simulink model "simulink_playground"  (R2019a)
settings: Solver=VariableStepAuto  StartTime=0.0  StopTime=0.1  MinStep=0.1  RelTol=1e-3
undefined symbols (not defined in the file or in its folder): MM
settings Model: Creator=carne  LastModifiedBy=carne
settings DataIOCC: ReturnWorkspaceOutputs=off
settings DebuggingCC: ArithmeticOperatorsInVariantConditions=warning

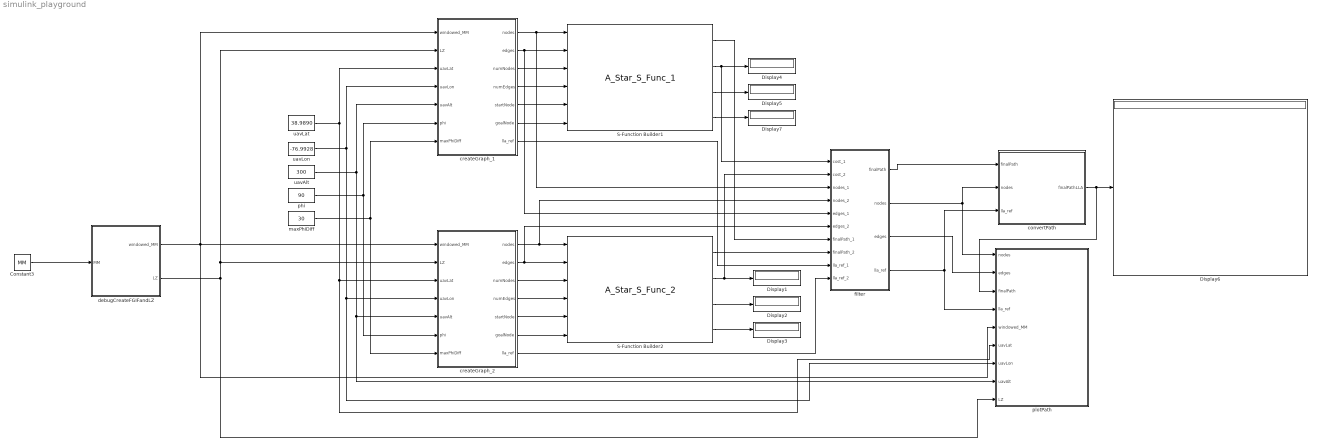
== system simulink_playground ==
  Constant3 : Constant  Value=MM
  Display{1..7} (7 alike) : Display
      Display1 settings: Format=decimal (Stored Integer)
      Display4 settings: Format=decimal (Stored Integer)
      Display6 settings: Format=decimal (Stored Integer)
  S-Function Builder1 : S-Function  InitFcn=try, set_param(gcb,'FunctionName','A_Star_S_Func_1'), end  FunctionName=A_Star_S_Func_1  SFunctionModules=A_Star_S_Func_1_wrapper  SFunctionDeploymentMode=off  EnableBusSupport=off  mask(S-Function Builder){}
      mask help: Simulink:masks:SFunctionBuilder_MD
      mask init:
      | val = [[.9  0.75 0.75 1 1 .9 .9 1]',[1 1 0.75 0.75 .9 .9 1 .9]'];try , sys = get_param(gcb,'SfunBuilderFcnName');if isempty(sys), sys = get_param(gcb,'FunctionName'); end,catch, sys = get_param(gcb,'FunctionName'); end
      settings: CopyFcn=set_param(gcbh,'LinkStatus','none')  PreSaveFcn=try, set_param(gcb,'FunctionName','A_Star_S_Func_1'), end  OpenFcn=sfunctionwizard(gcbh)
      mask Display: plot(val(:,1),val(:,2)),disp(sys), port_label('input',1,'nodeArray'), port_label('input',2,'edgeArray'), port_label('input',3,'numNodesPtr'), port_label('input',4,'numEdgesPtr'), port_label('input',5,'startNodePtr'), port_label('input',6,'goalNodePtr'), port_label('output',1,'finalPath'), port_label('output',2,'finalPathCost'), port_label('output',3,'numNodesCheck'), port_label('output',4,'numEdgesCheck')
  S-Function Builder2 : S-Function  InitFcn=try, set_param(gcb,'FunctionName','A_Star_S_Func_2'), end  FunctionName=A_Star_S_Func_2  SFunctionModules=A_Star_S_Func_2_wrapper  SFunctionDeploymentMode=off  EnableBusSupport=off  mask(S-Function Builder){}
      mask help: Simulink:masks:SFunctionBuilder_MD
      mask init: same as simulink_playground/S-Function Builder1
      settings: CopyFcn=set_param(gcbh,'LinkStatus','none')  PreSaveFcn=try, set_param(gcb,'FunctionName','A_Star_S_Func_2'), end  OpenFcn=sfunctionwizard(gcbh)
      mask Display: plot(val(:,1),val(:,2)),disp(sys), port_label('input',1,'nodeArray'), port_label('input',2,'edgeArray'), port_label('input',3,'numNodesPtr'), port_label('input',4,'numEdgesPtr'), port_label('input',5,'startNodePtr'), port_label('input',6,'goalNodePtr'), port_label('output',1,'finalPath'), port_label('output',2,'finalPathCost'), port_label('output',3,'numNodesCheck'), port_label('output',4,'numEdgesCheck')
  convertPath : MATLAB Function  TreatAsAtomicUnit=on
  createGraph_1 : MATLAB Function  TreatAsAtomicUnit=on
  createGraph_2 : MATLAB Function  TreatAsAtomicUnit=on
  debugCreateFGIFandLZ : MATLAB Function  TreatAsAtomicUnit=on
  filter : MATLAB Function  TreatAsAtomicUnit=on
  maxPhiDiff : Constant  Value=30
  phi : Constant  Value=90
  plotPath : MATLAB Function  TreatAsAtomicUnit=on
  uavAlt : Constant  Value=300
  uavLat : Constant  Value=38.9890
  uavLon : Constant  Value=-76.9928
  wires:
  createGraph_1/4(numEdges) -> S-Function Builder1/4
  createGraph_1/3(numNodes) -> S-Function Builder1/3
  createGraph_1/1(nodes) -> filter/3(nodes_1), S-Function Builder1/1
  createGraph_1/2(edges) -> filter/5(edges_1), S-Function Builder1/2
  S-Function Builder1/3 -> Display5/1
  S-Function Builder1/2 -> filter/1(cost_1), Display4/1
  uavAlt/1 -> plotPath/8(uavAlt), createGraph_2/5(uavAlt), createGraph_1/5(uavAlt)
  Constant3/1 -> debugCreateFGIFandLZ/1(MM)
  debugCreateFGIFandLZ/2(LZ) -> createGraph_1/2(LZ), createGraph_2/2(LZ), plotPath/9(LZ)
  S-Function Builder1/4 -> Display7/1
  uavLon/1 -> plotPath/7(uavLon), createGraph_2/4(uavLon), createGraph_1/4(uavLon)
  uavLat/1 -> plotPath/6(uavLat), createGraph_2/3(uavLat), createGraph_1/3(uavLat)
  phi/1 -> createGraph_2/6(phi), createGraph_1/6(phi)
  maxPhiDiff/1 -> createGraph_2/7(maxPhiDiff), createGraph_1/7(maxPhiDiff)
  convertPath/1(finalPathLLA) -> plotPath/3(finalPath), Display6/1
  debugCreateFGIFandLZ/1(windowed_MM) -> plotPath/5(windowed_MM), createGraph_1/1(windowed_MM), createGraph_2/1(windowed_MM)
  createGraph_1/5(startNode) -> S-Function Builder1/5
  createGraph_1/6(goalNode) -> S-Function Builder1/6
  createGraph_2/4(numEdges) -> S-Function Builder2/4
  createGraph_2/3(numNodes) -> S-Function Builder2/3
  createGraph_2/2(edges) -> filter/6(edges_2), S-Function Builder2/2
  createGraph_2/1(nodes) -> filter/4(nodes_2), S-Function Builder2/1
  createGraph_2/5(startNode) -> S-Function Builder2/5
  createGraph_2/6(goalNode) -> S-Function Builder2/6
  S-Function Builder2/3 -> Display2/1
  S-Function Builder2/2 -> filter/2(cost_2), Display1/1
  S-Function Builder2/4 -> Display3/1
  filter/1(finalPath) -> convertPath/1(finalPath)
  filter/2(nodes) -> convertPath/2(nodes), plotPath/1(nodes)
  filter/4(lla_ref) -> convertPath/3(lla_ref), plotPath/4(lla_ref)
  filter/3(edges) -> plotPath/2(edges)
  S-Function Builder2/1 -> filter/8(finalPath_2)
  S-Function Builder1/1 -> filter/7(finalPath_1)
  createGraph_2/7(lla_ref) -> filter/10(lla_ref_2)
  createGraph_1/7(lla_ref) -> filter/9(lla_ref_1)

== matlab function simulink_playground/plotPath ==
  data: nodes input; edges input; finalPath input; lla_ref input; windowed_MM input; uavLat input; uavLon input; uavAlt input; LZ input
function plotPath(nodes, edges, finalPath, lla_ref, windowed_MM, uavLat, uavLon, uavAlt, LZ)

    % setup altitude array for 3D matrix
    altDelta = 20.0;
    
    % convert altitude to meters
    uavAlt = uavAlt * 0.3048; % convert alt to meters
    altDelta = altDelta * 0.3048; % convert to meters
    
    % instantiate goal node variables
    goalNode = 0;
    goalNodeRow = 0;
    goalNodeCol = 0;
    
    numLzRows = max(LZ(:,1)) - min(LZ(:,1)) + 1;
    numLzCols = max(LZ(:,2)) - min(LZ(:,2)) + 1;
    
    % set the goal node row and column based on the orientation of the LZ
    if numLzRows > numLzCols
        goalNodeRow = min(LZ(:,1)); % right now pick one end of the LZ
        goalNodeCol = min(LZ(:,2)) + floor(numLzCols / 2); % pick the center column
    elseif numLzRows < numLzCols
        goalNodeCol = min(LZ(:,2)); % right now pick one end of the LZ
        goalNodeRow = min(LZ(:,1)) + floor(numLzRows / 2); % pick the center column
    end
    
    %% Create Altitude Array
    
    % setup altitude array for 3D matrix
    % currently this goes from UAV alt to zero, need to update this to
    % limit the lower altitude to the elevation of the landing strip
%     lzAlt = windowed_MM(goalNodeRow, goalNodeCol, 2);
%     altArray = [uavAlt:-altDelta:lzAlt];
%     if altArray(end) > lzAlt
%         altArray = [altArray, lzAlt];
%     end
%     [~, heightNum] = size(altArray);

    % WGS84 ellipsoid constants:
    a = 6378137;
    e = 8.1819190842622e-2;
    
    windowed_MM(:,:,4) = windowed_MM(:,:,4)==10000;

    reducedNodes = nodes(any(nodes,2),:);
    reducedEdges = edges(any(edges,2),:);

    coder.extrinsic('plot')
    coder.extrinsic('scatter')
    coder.extrinsic('plot3')
    coder.extrinsic('scatter3')

    close all
    figure()
    hold on
%    scatter3(reducedNodes(:,2),reducedNodes(:,3),reducedNodes(:,4),'filled','s')
%     for i = 1:length(reducedEdges(:,1))
%         x = [reducedNodes(reducedEdges(i,1),2),reducedNodes(reducedEdges(i,2),2)];
%         y = [reducedNodes(reducedEdges(i,1),3),reducedNodes(reducedEdges(i,2),3)];
%         z = [reducedNodes(reducedEdges(i,1),4),reducedNodes(reducedEdges(i,2),4)];
%         plot3(x,y,z,'r-');
%     end
    
     lat_ref = lla_ref(1);
     lon_ref = lla_ref(2);
     alt_ref = lla_ref(3);

    %reducedFinalPath = finalPath(finalPath ~= 0);
    %plot3(reducedNodes(reducedFinalPath',2),reducedNodes(reducedFinalPath',3),reducedNodes(reducedFinalPath',4),'g*-','LineWidth',2);
    
    reducedFinalPathLLA = finalPath(finalPath(:,1) ~= 0,:);
    reducedFinalPathENU = zeros(length(reducedFinalPathLLA(:,1)),3);
    
    for i = 1:length(reducedFinalPathLLA(:,1))
        lat = reducedFinalPathLLA(i,1);
        lon = reducedFinalPathLLA(i,2);
        alt = reducedFinalPathLLA(i,3);
        
        [east,north,up] = lla2enu(lat,lon,alt,lat_ref,lon_ref,alt_ref);
        
        reducedFinalPathENU(i,:) = [east,north,up];
        
    end
    
    plot3(reducedFinalPathENU(:,1),reducedFinalPathENU(:,2),reducedFinalPathENU(:,3),'g*-','LineWidth',2);
    
    
    %plot3(reducedNodes(reducedFinalPath(end),2),reducedNodes(reducedFinalPath(end),3),reducedNodes(reducedFinalPath(end),4),'g^','MarkerSize',10,'MarkerFaceColor','g');
    [rowCount, colCount] = size(windowed_MM(:,:,1));
    
    % convert UAV position to ENU
    [uavE,uavN,uavU] = lla2enu(uavLat,uavLon,uavAlt,lat_ref,lon_ref,alt_ref);
    
    % plot actual UAV position
    plot3(uavE,uavN,uavU,'g^','MarkerSize',10,'MarkerFaceColor','g');
    
    trimmed_MM_enu = zeros (rowCount, colCount, 3);
    
    for i = 1:rowCount
        for j = 1:colCount
            lon = windowed_MM(i, j, 5);
            lat = windowed_MM(i, j, 6);
            alt = windowed_MM(i, j, 2);
            
            [e,n,u] = lla2enu(lat,lon,alt,lat_ref,lon_ref,alt_ref);
            trimmed_MM_enu(i, j, 1) = e;
            trimmed_MM_enu(i, j, 2) = n;
            trimmed_MM_enu(i, j, 3) = u;
        end
    end
    
    mesh(trimmed_MM_enu(:,:,1), trimmed_MM_enu(:,:,2), trimmed_MM_enu(:,:,3));
    
    for i = 1:rowCount
        for j = 1:colCount
            if (windowed_MM(i,j,4))
                
                % intermediate calcs for conversion to ECEF
                lat = windowed_MM(i, j, 6);
                lon = windowed_MM(i, j, 5);
                alt = windowed_MM(i,j,2) + 0.5;

                % convert to ENU
                [e,n,u] = lla2enu(lat,lon,alt,lat_ref,lon_ref,alt_ref);

                plot3(e,n,u,'rs','MarkerSize',4,'MarkerFaceColor','r');
            end
        end
    end
    
    for i = 1:length(LZ(:,1))
        plot3(trimmed_MM_enu(LZ(i,1),LZ(i,2),1),...
            trimmed_MM_enu(LZ(i,1),LZ(i,2),2),...
            trimmed_MM_enu(LZ(i,1),LZ(i,2),3),...
            'bs','MarkerSize',4,'MarkerFaceColor','b');
    end
    
    xlabel('ENU East (m)')
    ylabel('ENU North (m)')
    zlabel('ENU Up (m)')
    
    
    stop = 1;

end

== matlab function simulink_playground/createGraph_1 ==
  data: nodes output; edges output; numNodes output; numEdges output; startNode output; windowed_MM input; LZ input; uavLat input; uavLon input; uavAlt input; phi input; maxPhiDiff input; goalNode output; lla_ref output
function [nodes, edges, numNodes, numEdges, startNode, goalNode, lla_ref] = createGraph(windowed_MM, LZ, uavLat, uavLon, uavAlt, phi, maxPhiDiff)
%% CREATEGRAPH: function to create the graph structure to feed to the A* algorithm
% NOTE: all input arguments should be immutable!

    % define the altitude delta (in meters) to use when constructing the
    % graph layers
    altDelta = 5.0; % meters

    % convert LS data to binary
    windowed_MM(:,:,4) = windowed_MM(:,:,4)==10000;
    
    % convert altitude to meters
    uavAlt = uavAlt * 0.3048; % convert to meters
    altDelta = altDelta * 0.3048; % convert to meters
    
    % instantiate variables to output
    nodes = zeros(1000000, 4);
    nodes_allInfo = zeros(1000000, 7);
    edges = zeros(1000000, 3);
    numEdges = 0;
    numNodes = 0;
    [rowNum, colNum, widthNum] = size(windowed_MM);
    nodeNum = rowNum * colNum;
    edgeNum = rowNum * colNum * 24 * 2;
    
    %% Determine Goal Node
    % set the goal node as one end of the landing strip
    
    % instantiate goal node variables
    goalNode = 0;
    goalNodeRow = 0;
    goalNodeCol = 0;
    
    numLzRows = max(LZ(:,1)) - min(LZ(:,1)) + 1;
    numLzCols = max(LZ(:,2)) - min(LZ(:,2)) + 1;
    
    % set the goal node row and column based on the orientation of the LZ
    if numLzRows > numLzCols
        goalNodeRow = min(LZ(:,1)); % right now pick one end of the LZ
        goalNodeCol = min(LZ(:,2)) + floor(numLzCols / 2); % pick the center column
    elseif numLzRows < numLzCols
        goalNodeCol = min(LZ(:,2)); % right now pick one end of the LZ
        goalNodeRow = min(LZ(:,1)) + floor(numLzRows / 2); % pick the center column
    end
    
    % set variables for conversion to ENU; save to export when we convert
    % back
    lat_ref = windowed_MM(goalNodeRow,goalNodeCol,6);
    lon_ref = windowed_MM(goalNodeRow,goalNodeCol,5);
    alt_ref = windowed_MM(goalNodeRow,goalNodeCol,2);
    lla_ref = [lat_ref,lon_ref,alt_ref];
    
    %% Determine Start Node
    
    % instantiate start node variables
    startNode = 0;
    
    % convert UAV LLA to ENU; we will select the closest node to use as the
    % start node as we create the node structure
    [uavE, uavN, uavU] = lla2enu(uavLat,uavLon,uavAlt,lat_ref,lon_ref,alt_ref);
    
    %% Create Altitude Array
    
    % setup altitude array for 3D matrix
    % currently this goes from UAV alt to zero, need to update this to
    % limit the lower altitude to the elevation of the landing strip
    lzAlt = windowed_MM(goalNodeRow, goalNodeCol, 2);
    altArray = [uavAlt:-altDelta:lzAlt];
    if altArray(end) > lzAlt
        altArray = [altArray, lzAlt];
    end
    [~, heightNum] = size(altArray);
    
    %% Populate Node Array
    
    % will also have a separate temporary node structure to hold all
    % applicable MM info for easy edge cost computing
    
    % will also check which node is the closest to the UAV current position
    % based on it's position and orientation
    
    % initialize difference variables used to get closest node
    startNodePosDiff = 1000000.0;
    startNodePosDiffTemp = 0.0;
    startNodeAngDiff = 0.0;
    
    % initialize variable to define the LZ approach nodes; these are the
    % nodes from which the goal node can be aproached and will be used when
    % generating the edges
    lzApproachNodes = [];
    
    for i = 1:rowNum
        for j = 1:colNum
            for h = 1:heightNum
                nodeEntry = ((i - 1) * colNum + (j - 1)) * heightNum + h;

                % convert to ENU
                alt = altArray(h);
                lat = windowed_MM(i, j, 6);
                lon = windowed_MM(i, j, 5);
                [e,n,u] = lla2enu(lat,lon,alt,lat_ref,lon_ref,alt_ref);

                % populate arrays
                nodes(nodeEntry, :) = [nodeEntry, e, n, u];
                nodes_allInfo(nodeEntry, :) = [nodeEntry, windowed_MM(i, j, 1), windowed_MM(i, j, 2), windowed_MM(i, j, 3), windowed_MM(i, j, 4), windowed_MM(i, j, 5), windowed_MM(i, j, 6)];
                
                % get goal node id
                if i == goalNodeRow && j == goalNodeCol && h == heightNum
                    goalNode = nodeEntry;
                end
                
                % add node to LZ approach nodes if applicable
                if (abs(i - goalNodeRow) < 2 && abs(j - goalNodeCol) < 2 &&...
                        ~ismember([i,j],LZ,'rows') && h == heightNum - 1)
                    lzApproachNodes = [nodeEntry, lzApproachNodes];
                end
                
                % if the current node is on the same level as the UAV,
                % check if it should be the startNode
                if alt == uavAlt
                    
                    % calculate angle difference (multiply by negative one
                    % to fit standard for measuring phi)
                    startNodeAngDiff = atan2(n - uavN, e - uavE);
                    
                    % convert -pi to pi measurement to zero to 2pi
                    if startNodeAngDiff < 0
                        startNodeAngDiff = startNodeAngDiff + 2 * pi;
                    end
                    
                    % convert to degrees
                    startNodeAngDiff = startNodeAngDiff * 180 / pi;
                    
                    % check if the current node is within the maximum
                    % search area set by the UAV's orientation
                    if abs(startNodeAngDiff - phi) <= maxPhiDiff
                        
                        % if the current node is closer than the selected
                        % start node, update the start node to the current
                        % node
                        startNodePosDiffTemp = hypot(n - uavN, e - uavE);
                        if startNodePosDiffTemp < startNodePosDiff
                            startNodePosDiff = startNodePosDiffTemp;
                            startNode = nodeEntry;
                        end
                    end
                end
            end
        end
    end

    %% Populate Edge Array
    
    % assume an 24-connected bidirectional 3D graph, but remove nodes that
    % would allow strictly vertical motion (not possible for fixed-wing)
    
    edgeEntryOffSet = 0;
    
    for i = 1:rowNum
        for j = 1:colNum
            for h = 1:heightNum 
                for k = 1:24
                    edgeEntry = (((i - 1) * colNum + (j - 1)) * heightNum + (h - 1)) * 24 + k - edgeEntryOffSet;

                    % determine height offset value
                    heightOffset = 0;
                    if ismember(k, [1:8])
                        heightOffset = 1;
                    elseif ismember(k, [17:24])
                        heightOffset = -1;
                    end
                    
                    % determine row offset value
                    rowOffset = 0;
                    if ismember(k, [1, 2, 3, 9, 10, 11, 17, 18, 19])
                        rowOffset = 1;
                    elseif ismember(k, [5, 6, 7, 13, 14, 15, 21, 22, 23])
                        rowOffset = -1;
                    end

                    % determine col offset value
                    colOffset = 0;
                    if ismember(k, [3, 4, 5, 11, 12, 13, 19, 20, 21])
                        colOffset = 1;
                    elseif ismember(k, [7, 8, 1, 15, 16, 9, 23, 24, 17])
                        colOffset = -1;
                    end

                    % define from and to nodes
                    fromNode = ((i - 1) * colNum + (j - 1)) * heightNum + h;
                    toNode = ((i + rowOffset- 1) * colNum + (j + colOffset - 1)) * heightNum + h + heightOffset;
                    
                    % if value of offset is outside of matrix, add to the offset
                    % value that is used to determine row position (essentially
                    % skipping that row in the order; else, populate the edge
                    % entry based on the iteration
                    if (i + rowOffset < 1 || i + rowOffset > rowNum ||...
                            j + colOffset < 1 || j + colOffset > colNum ||...
                            h + heightOffset < 1 || h + heightOffset > heightNum ||...
                            (toNode == goalNode && ~ismember(fromNode, lzApproachNodes)))
                        edgeEntryOffSet = edgeEntryOffSet + 1;
                    else

                        % set initial cost
                        cost = 100;
    
                        % determine 2-norm of difference vector and add to
                        % cost
                        diffVect = [
                            nodes(toNode,2) - nodes(fromNode,2),
                            nodes(toNode,3) - nodes(fromNode,3),
                            nodes(toNode,4) - nodes(fromNode,4)
                            ];
                        cost = cost + norm(diffVect);
                        
                        % add cost to edges that lead to a node closer to
                        % the ground
                        nodeAlt = uavAlt - (h + heightOffset) * altDelta; % the altitude of the toNode
                        distToGround = nodeAlt - nodes_allInfo(toNode,3);
                        if distToGround > 0
                            cost = cost + 100 * (1.0 - distToGround / uavAlt);
                        else
                            cost = cost + 10000;
                        end
                        
                        % if edge leads to a higher node (i.e. gains
                        % altitude) add cost; this could change depending
                        % on the fault mode
                        if heightOffset > 0
                            cost = cost + 10000;
                        end

                        % if the edge goes to a node over a populated
                        % region, add to the cost
                        if (nodes_allInfo(toNode,5))
                            cost = cost + 5000;
                        end

                        edges(edgeEntry, :) = [fromNode, toNode, cost];
                    end
                end
            end
        end
    end

    %% Wrap-Up
    % export the number of nodes and edges as a sanity check for the A*
    % algo runs
    
    numNodes = nnz(nodes(:,1));
    numEdges = nnz(edges(:,1));

    end

== matlab function simulink_playground/debugCreateFGIFandLZ ==
  data: MM input; windowed_MM output; LZ output
function [windowed_MM, LZ] = debugCreateVars(MM)

    %windowed_MM = MM(26:50,26:35,:);
    windowed_MM = MM(1:50,1:35,:);
    LZ = zeros(15,2);
    
    LZ(1:5,:) = [[19:23]',ones(5,1)*1];
    LZ(6:10,:) = [[19:23]',ones(5,1)*2];
    LZ(11:15,:) = [[19:23]',ones(5,1)*3];
    
    %LZ = windowed_MM(1:5,1:3);

end

== matlab function simulink_playground/convertPath ==
  data: finalPath input; finalPathLLA output; nodes input; lla_ref input
function finalPathLLA = convertPath(finalPath, nodes, lla_ref)
%% Path Conversion and ENU Array Generation

    % extract just the nonzero entries from the final path array
    reducedFinalPath = flip(finalPath(finalPath ~= 0));
    [~,numCols] = size(reducedFinalPath);
    
    % instantiate variable
    finalPathLLA_trimmed = zeros(1000000, 3);
    finalPathLLA = zeros(1000000, 3);
    finalPathENU = zeros(1000000, 3);

    for i = 1:numCols
       % get the ENU coordinates from the nodes array
       east = nodes(reducedFinalPath(i),2);
       north = nodes(reducedFinalPath(i),3);
       up = nodes(reducedFinalPath(i),4);

       % populate ENU array
       finalPathENU(i,:) = [east,north,up];
       
       % convert to LLA
       [lat,lon,alt] = enu2lla(east, north, up, lla_ref(1), lla_ref(2), lla_ref(3));

       % populate LLA array
       finalPathLLA(i,:) = [lat,lon,alt];
    end

%% Point Removal
% use 3D linear interpolation to remove points on the same line

    finalPathLLA_trimmed(1,:) = finalPathLLA(1,:);
    finalPointCount = 1;

    for i = 3:length(finalPathENU(:,1))

        % set points
        p1 = [finalPathENU(i - 2,1),finalPathENU(i - 2,2),finalPathENU(i - 2,3)];
        p2 = [finalPathENU(i - 1,1),finalPathENU(i - 1,2),finalPathENU(i - 1,3)];
        p3 = [finalPathENU(i,1),finalPathENU(i,2),finalPathENU(i,3)];

        % determine difference vectors
        v1 = p3 - p1;
        v2 = p3 - p2;

        % check if vector norms are equivalent, if not, keep point in final
        % path
        n1 = v1 / norm(v1);
        n2 = v2 / norm(v2);

        if norm(n1 - n2) > 0.001
            finalPointCount = finalPointCount + 1;
            finalPathLLA_trimmed(finalPointCount,:) = finalPathLLA(i,:);
        end

    end    
    
    finalPathLLA = finalPathLLA_trimmed;
    
    test = 1;
    
end

== matlab function simulink_playground/createGraph_2 ==
  data: nodes output; edges output; numNodes output; numEdges output; startNode output; windowed_MM input; LZ input; uavLat input; uavLon input; uavAlt input; phi input; maxPhiDiff input; goalNode output; lla_ref output
function [nodes, edges, numNodes, numEdges, startNode, goalNode, lla_ref] = createGraph(windowed_MM, LZ, uavLat, uavLon, uavAlt, phi, maxPhiDiff)
%% CREATEGRAPH: function to create the graph structure to feed to the A* algorithm
% NOTE: all input arguments should be immutable!

    % define the altitude delta (in meters) to use when constructing the
    % graph layers
    altDelta = 5.0; % meters

    % convert LS data to binary
    windowed_MM(:,:,4) = windowed_MM(:,:,4)==10000;
    
    % convert altitude to meters
    uavAlt = uavAlt * 0.3048; % convert to meters
    altDelta = altDelta * 0.3048; % convert to meters
    
    % instantiate variables to output
    nodes = zeros(1000000, 4);
    nodes_allInfo = zeros(1000000, 7);
    edges = zeros(1000000, 3);
    numEdges = 0;
    numNodes = 0;
    [rowNum, colNum, widthNum] = size(windowed_MM);
    nodeNum = rowNum * colNum;
    edgeNum = rowNum * colNum * 24 * 2;
    
    %% Determine Goal Node
    % set the goal node as one end of the landing strip
    
    % instantiate goal node variables
    goalNode = 0;
    goalNodeRow = 0;
    goalNodeCol = 0;
    
    numLzRows = max(LZ(:,1)) - min(LZ(:,1)) + 1;
    numLzCols = max(LZ(:,2)) - min(LZ(:,2)) + 1;
    
    % set the goal node row and column based on the orientation of the LZ
    if numLzRows > numLzCols
        goalNodeRow = max(LZ(:,1)); % right now pick one end of the LZ
        goalNodeCol = min(LZ(:,2)) + floor(numLzCols / 2); % pick the center column
    elseif numLzRows < numLzCols
        goalNodeCol = max(LZ(:,2)); % right now pick one end of the LZ
        goalNodeRow = min(LZ(:,1)) + floor(numLzRows / 2); % pick the center column
    end
    
    % set variables for conversion to ENU; save to export when we convert
    % back
    lat_ref = windowed_MM(goalNodeRow,goalNodeCol,6);
    lon_ref = windowed_MM(goalNodeRow,goalNodeCol,5);
    alt_ref = windowed_MM(goalNodeRow,goalNodeCol,2);
    lla_ref = [lat_ref,lon_ref,alt_ref];
    
    %% Determine Start Node
    
    % instantiate start node variables
    startNode = 0;
    
    % convert UAV LLA to ENU; we will select the closest node to use as the
    % start node as we create the node structure
    [uavE, uavN, uavU] = lla2enu(uavLat,uavLon,uavAlt,lat_ref,lon_ref,alt_ref);
    
    %% Create Altitude Array
    
    % setup altitude array for 3D matrix
    % currently this goes from UAV alt to zero, need to update this to
    % limit the lower altitude to the elevation of the landing strip
    lzAlt = windowed_MM(goalNodeRow, goalNodeCol, 2);
    altArray = [uavAlt:-altDelta:lzAlt];
    if altArray(end) > lzAlt
        altArray = [altArray, lzAlt];
    end
    [~, heightNum] = size(altArray);
    
    %% Populate Node Array
    
    % will also have a separate temporary node structure to hold all
    % applicable MM info for easy edge cost computing
    
    % will also check which node is the closest to the UAV current position
    % based on it's position and orientation
    
    % initialize difference variables used to get closest node
    startNodePosDiff = 1000000.0;
    startNodePosDiffTemp = 0.0;
    startNodeAngDiff = 0.0;
    
    % initialize variable to define the LZ approach nodes; these are the
    % nodes from which the goal node can be aproached and will be used when
    % generating the edges
    lzApproachNodes = [];
    
    for i = 1:rowNum
        for j = 1:colNum
            for h = 1:heightNum
                nodeEntry = ((i - 1) * colNum + (j - 1)) * heightNum + h;

                % convert to ENU
                alt = altArray(h);
                lat = windowed_MM(i, j, 6);
                lon = windowed_MM(i, j, 5);
                [e,n,u] = lla2enu(lat,lon,alt,lat_ref,lon_ref,alt_ref);

                % populate arrays
                nodes(nodeEntry, :) = [nodeEntry, e, n, u];
                nodes_allInfo(nodeEntry, :) = [nodeEntry, windowed_MM(i, j, 1), windowed_MM(i, j, 2), windowed_MM(i, j, 3), windowed_MM(i, j, 4), windowed_MM(i, j, 5), windowed_MM(i, j, 6)];
                
                % get goal node id
                if i == goalNodeRow && j == goalNodeCol && h == heightNum
                    goalNode = nodeEntry;
                end
                
                % add node to LZ approach nodes if applicable
                if (abs(i - goalNodeRow) < 2 && abs(j - goalNodeCol) < 2 &&...
                        ~ismember([i,j],LZ,'rows') && h == heightNum - 1)
                    lzApproachNodes = [nodeEntry, lzApproachNodes];
                end
                
                % if the current node is on the same level as the UAV,
                % check if it should be the startNode
                if alt == uavAlt
                    
                    % calculate angle difference (multiply by negative one
                    % to fit standard for measuring phi)
                    startNodeAngDiff = atan2(n - uavN, e - uavE);
                    
                    % convert -pi to pi measurement to zero to 2pi
                    if startNodeAngDiff < 0
                        startNodeAngDiff = startNodeAngDiff + 2 * pi;
                    end
                    
                    % convert to degrees
                    startNodeAngDiff = startNodeAngDiff * 180 / pi;
                    
                    % check if the current node is within the maximum
                    % search area set by the UAV's orientation
                    if abs(startNodeAngDiff - phi) <= maxPhiDiff
                        
                        % if the current node is closer than the selected
                        % start node, update the start node to the current
                        % node
                        startNodePosDiffTemp = hypot(n - uavN, e - uavE);
                        if startNodePosDiffTemp < startNodePosDiff
                            startNodePosDiff = startNodePosDiffTemp;
                            startNode = nodeEntry;
                        end
                    end
                end
            end
        end
    end

    %% Populate Edge Array
    
    % assume an 24-connected bidirectional 3D graph, but remove nodes that
    % would allow strictly vertical motion (not possible for fixed-wing)
    
    edgeEntryOffSet = 0;
    
    for i = 1:rowNum
        for j = 1:colNum
            for h = 1:heightNum 
                for k = 1:24
                    edgeEntry = (((i - 1) * colNum + (j - 1)) * heightNum + (h - 1)) * 24 + k - edgeEntryOffSet;

                    % determine height offset value
                    heightOffset = 0;
                    if ismember(k, [1:8])
                        heightOffset = 1;
                    elseif ismember(k, [17:24])
                        heightOffset = -1;
                    end
                    
                    % determine row offset value
                    rowOffset = 0;
                    if ismember(k, [1, 2, 3, 9, 10, 11, 17, 18, 19])
                        rowOffset = 1;
                    elseif ismember(k, [5, 6, 7, 13, 14, 15, 21, 22, 23])
                        rowOffset = -1;
                    end

                    % determine col offset value
                    colOffset = 0;
                    if ismember(k, [3, 4, 5, 11, 12, 13, 19, 20, 21])
                        colOffset = 1;
                    elseif ismember(k, [7, 8, 1, 15, 16, 9, 23, 24, 17])
                        colOffset = -1;
                    end

                    % define from and to nodes
                    fromNode = ((i - 1) * colNum + (j - 1)) * heightNum + h;
                    toNode = ((i + rowOffset- 1) * colNum + (j + colOffset - 1)) * heightNum + h + heightOffset;
                    
                    % if value of offset is outside of matrix, add to the offset
                    % value that is used to determine row position (essentially
                    % skipping that row in the order; else, populate the edge
                    % entry based on the iteration
                    if (i + rowOffset < 1 || i + rowOffset > rowNum ||...
                            j + colOffset < 1 || j + colOffset > colNum ||...
                            h + heightOffset < 1 || h + heightOffset > heightNum ||...
                            (toNode == goalNode && ~ismember(fromNode, lzApproachNodes)))
                        edgeEntryOffSet = edgeEntryOffSet + 1;
                    else

                        % set initial cost
                        cost = 100;
    
                        % determine 2-norm of difference vector and add to
                        % cost
                        diffVect = [
                            nodes(toNode,2) - nodes(fromNode,2),
                            nodes(toNode,3) - nodes(fromNode,3),
                            nodes(toNode,4) - nodes(fromNode,4)
                            ];
                        cost = cost + norm(diffVect);
                        
                        % add cost to edges that lead to a node closer to
                        % the ground
                        nodeAlt = uavAlt - (h + heightOffset) * altDelta; % the altitude of the toNode
                        distToGround = nodeAlt - nodes_allInfo(toNode,3);
                        if distToGround > 0
                            cost = cost + 100 * (1.0 - distToGround / uavAlt);
                        else
                            cost = cost + 10000;
                        end
                        
                        % if edge leads to a higher node (i.e. gains
                        % altitude) add cost; this could change depending
                        % on the fault mode
                        if heightOffset > 0
                            cost = cost + 10000;
                        end

                        % if the edge goes to a node over a populated
                        % region, add to the cost
                        if (nodes_allInfo(toNode,5))
                            cost = cost + 5000;
                        end

                        edges(edgeEntry, :) = [fromNode, toNode, cost];
                    end
                end
            end
        end
    end

    %% Wrap-Up
    % export the number of nodes and edges as a sanity check for the A*
    % algo runs
    
    numNodes = nnz(nodes(:,1));
    numEdges = nnz(edges(:,1));

    end

== matlab function simulink_playground/filter ==
  data: finalPath output; cost_1 input; nodes output; cost_2 input; nodes_1 input; nodes_2 input; edges_1 input; edges_2 input; finalPath_1 input; finalPath_2 input; lla_ref_1 input; lla_ref_2 input; edges output; lla_ref output
function [finalPath, nodes, edges, lla_ref] = filter(cost_1, cost_2, nodes_1, nodes_2, edges_1, edges_2, finalPath_1, finalPath_2, lla_ref_1, lla_ref_2)

%% Path Selection
% determine which set of points to use based on cost

    nodes = nodes_1;
    edges = edges_1;
    finalPath = finalPath_1;
    lla_ref = lla_ref_1;
    
    if cost_1 > cost_2
        nodes = nodes_2;
        edges = edges_2;
        finalPath = finalPath_2;
        lla_ref = lla_ref_2;
    end

end
